simulink model "PID"  (R2020b)
settings: Solver=VariableStepAuto  StartTime=0.0  StopTime=300.0  RelTol=1e-3
values from neighbouring files (symbols this model uses):
  Kp = (0.9*T0)/(K0*(tau + 0.5*T)) - (0.5*Ki)/K0    (= 0.670050069403)    [Parametri_PI.m]    (also in Parametri_PID.m = 0.886775962404)
  T = 0.01    [Parametri_PI.m]    (also in Parametri_PID.m)
  Td = 0    [Parametri_PI.m]    (also in Parametri_PID.m = 0.310112149696)
  Ti = (Kp*T)/Ki    (= 2.4575)    [Parametri_PI.m]    (also in Parametri_PID.m = 1.46356729475)
libraries: simulink x1
settings Model: Creator=user  LastModifiedBy=user

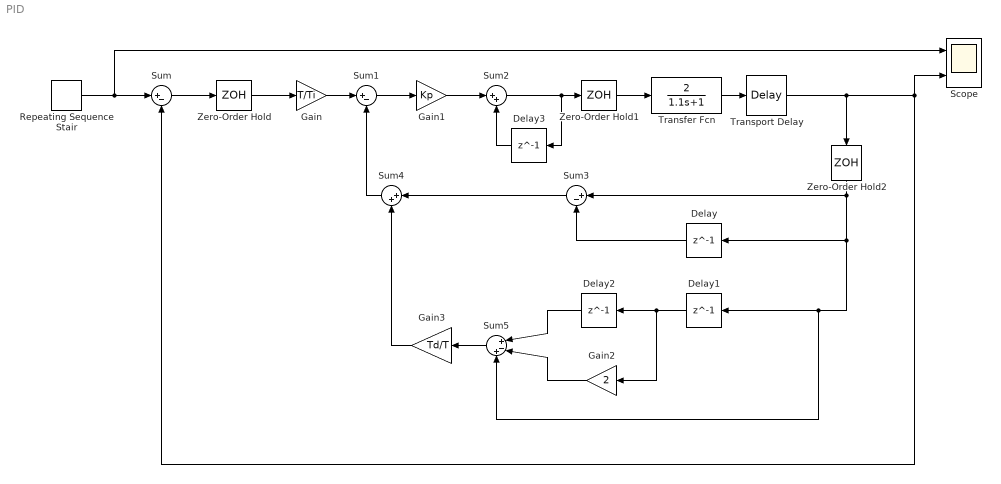
== system PID ==
  Delay{,1..3} (4 alike) : Delay  DelayLength=1
  Gain : Gain  Gain=T/Ti
  Gain1 : Gain  Gain=Kp
  Gain2 : Gain  Gain=2
  Gain3 : Gain  Gain=Td/T
  Repeating Sequence Stair : simulink/Sources/Repeating Sequence Stair  OutValues=[3 1 -5 2 1].'  tsamp=50  OutMin=[]  OutMax=[]  OutDataTypeStr=double  OutputDataTypeScalingMode=double  OutDataType=fixdt(0,8)  ConRadixGroup=Best Precision: Vector-wise  OutScaling=2^-12
  Scope : Scope  NumInputPorts=2
  Sum : Sum  Inputs=|+-
  Sum1 : Sum  Inputs=|+-
  Sum2 : Sum  Inputs=|++
  Sum3 : Sum  Inputs=|+-
  Sum4 : Sum  Inputs=|++
  Sum5 : Sum  Inputs=|+-+
  Transfer Fcn : TransferFcn  Numerator=[2]  Denominator=[1.1 1]
  Transport Delay : TransportDelay  DelayTime=0.773
  Zero-Order Hold : ZeroOrderHold  SampleTime=0.01
  Zero-Order Hold1 : ZeroOrderHold  SampleTime=0.01
  Zero-Order Hold2 : ZeroOrderHold  SampleTime=0.01
  wires:
  Sum5/1 -> Gain3/1
  Gain1/1 -> Sum2/1
  Sum1/1 -> Gain1/1
  Sum2/1 -> Delay3/1, Zero-Order Hold1/1
  Gain/1 -> Sum1/1
  Transfer Fcn/1 -> Transport Delay/1
  Delay1/1 -> Gain2/1, Delay2/1
  Gain3/1 -> Sum4/2
  Delay2/1 -> Sum5/1
  Delay3/1 -> Sum2/2
  Zero-Order Hold2/1 -> Sum5/3, Delay1/1, Delay/1, Sum3/1
  Delay/1 -> Sum3/2
  Sum/1 -> Zero-Order Hold/1
  Zero-Order Hold/1 -> Gain/1
  Gain2/1 -> Sum5/2
  Transport Delay/1 -> Sum/2, Scope/2, Zero-Order Hold2/1
  Repeating Sequence Stair/1 -> Scope/1, Sum/1
  Sum4/1 -> Sum1/2
  Zero-Order Hold1/1 -> Transfer Fcn/1
  Sum3/1 -> Sum4/1
